simulink model "stateMachine"  (R2021a)
settings: Solver=VariableStepAuto  StartTime=0.0  StopTime=inf  RelTol=1e-3
libraries: vrlib x1
settings Model: Creator=Al ien  LastModifiedBy=Al ien

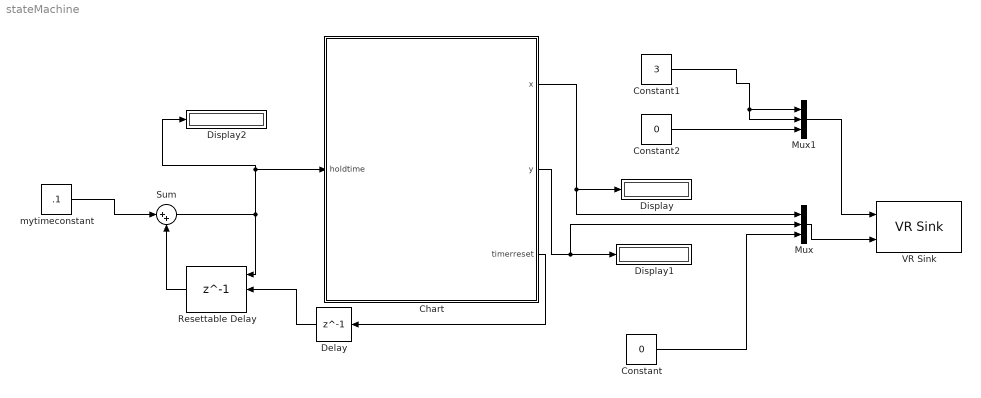
== system stateMachine ==
  Chart : Stateflow chart  TreatAsAtomicUnit=on
  Constant : Constant  Value=0
  Constant1 : Constant  Value=3
  Constant2 : Constant  Value=0
  Delay : Delay  DelayLength=1  InitialCondition=0
  Display : Display
  Display1 : Display
  Display2 : Display
  Mux : Mux  Inputs=3
  Mux1 : Mux  Inputs=3
  Resettable Delay : Delay  DelayLength=1  InitialConditionSource=Input port  ExternalReset=Rising
      settings: InputPortMap=u0,r5,p4
  Sum : Sum  Inputs=|++
  VR Sink : vrlib/VR Sink  InstantiateOnLoad=on  SampleTime=0.1  ViewEnable=on  RemoteChange=off  RemoteView=off  FieldsWritten=outer.translation.3.1.1.double#cursor.translation.3.1.1.double  WorldFileName=C:\Users\Al ien\Documents\spheres.WRL  AutoView=off  VideoDimensions=[]  AllowVariableSize=off  FigureProperties="{'Position', 'Name', 'Viewpoint', 'CameraBound', 'CameraDirection', 'CameraPosition', 'CameraUpVector', 'ZoomFactor', 'Antialiasing', 'Headlight', 'Lighting', 'NavPanel', 'Sound', 'StatusBar', 'Stereo3D', 'Stereo3DCameraOffset', 'Stereo3DHIT', 'ToolBar', 'Textures', 'Transparency', 'Triad', 'Wireframe', 'NavZones', 'NavMode', 'NavSpeed', 'CaptureFileFormat', 'CaptureFileName', 'Record2DCompressMethod', 'Record2DCompressQuality', 'Record2D', 'Record2DFileName', 'Record2DFPS'; [5.4500000000000000e+01   5.4400000000000000e+02   5.7600000000000000e+02   3.5000000000000000e+02], '', '', 'on', [6.1015813584369270e-02   3.1410759078128521e-02  -9.9764243830482069e-01], [-1.4121662559160091e+00   8.7394714355468750e-03   1.3469981744589880e+01], [-1.9174991905538939e-03   9.9950656036573160e-01   3.1352176682304597e-02], [1.0000000000000000e+00], 'on', 'on', 'on', 'halfbar', 'on', 'on', 'off', [1.0000000149011612e-01], [0.0000000000000000e+00], 'on', 'on', 'on', 'none', 'off', 'off', 'fly', 'normal', 'tif', '%f_anim_%n.tif', 'auto', [7.5000000000000000e+01], 'off', '%f_anim_%n.avi', 'auto'}"
  mytimeconstant : Constant  Value=.1
  wires:
  Chart/2(y) -> Mux/2, Display1/1
  Chart/1(x) -> Mux/1, Display/1
  Sum/1 -> Display2/1, Chart/1(holdtime), Resettable Delay/1
  mytimeconstant/1 -> Sum/1
  Resettable Delay/1 -> Sum/2
  Chart/3(timerreset) -> Delay/1
  Delay/1 -> Resettable Delay/2
  Constant/1 -> Mux/3
  Mux/1 -> VR Sink/2
  Constant1/1 -> Mux1/2, Mux1/1
  Constant2/1 -> Mux1/3
  Mux1/1 -> VR Sink/1

== stateflow chart stateMachine/Chart ==
  state startstate
    x=0; y=0; timerreset=0;
  state resettimerstate
    x=0; y=0; timerreset=1;
  state centerstate
    x=0; y=0; timerreset=0;
  state outerstatetransition
    x=x+0.01; y=y+0.01; timerreset=0;
  state centerstateback
    x=0; y=0; timerreset=0;
  state outerstate
    x=3; y=3; timerreset=0;
  state centerstatetransition
    x=x-0.01; y=y-0.01; timerreset=0;
  (default) -> startstate
  startstate -> centerstate
  resettimerstate -> centerstate
  centerstateback -> resettimerstate : [holdtime>150]
  centerstate -> outerstatetransition : [holdtime>25]
  outerstatetransition -> outerstate : [x>=3 && y>= 3]
  centerstatetransition -> centerstateback : [x<=0 && y<=0]
  outerstate -> centerstatetransition : [holdtime>100]
  data: x output; y output; holdtime input; timerreset output
